simulink model "astrobotics_flowchart"  (R2018a)
settings: Solver=FixedStepDiscrete  StartTime=0.0  StopTime=60  FixedStep=0.1  RelTol=1e-3  EnableMultiTasking=on
settings Model: Creator=alex  LastModifiedBy=alex
settings SolverCC: AutoInsertRateTranBlk=on
settings DataIOCC: LimitDataPoints=on
settings OptimizationCC: LifeSpan=inf
settings DebuggingCC: AllowSymbolicDim=off  SFUnexpectedBacktrackingDiag=warning  SFNoUnconditionalDefaultTransitionDiag=warning  SFExecutionAtInitializationDiag=none
settings CodeAppCC: StateflowObjectComments=on
settings GRTTargetCC: TargetLangStandard=C89/C90 (ANSI)
settings ConfigComp: CovMetricSettings=dw  CovHtmlReporting=on  CovSaveCumulativeToWorkspaceVar=on  CovSaveSingleToWorkspaceVar=on  CovShowResultsExplorer=off  CovExternalEMLEnable=off

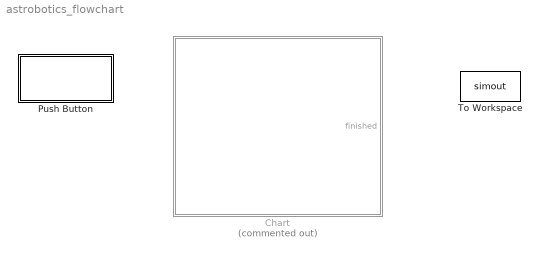
== system astrobotics_flowchart ==
  Chart : Stateflow chart  Commented=on  TreatAsAtomicUnit=on
  Push Button : Subsystem  DialogController=hmiCreateDDGDialog  IsWebBlock=on  mask(MWDashboardBlock){webBlockId=0eb19dcc-6111-4502-8404-cb3df8c1d0d6, webBlockType=pushbutton, ShowInLibBrwoser=on, ShowInitialText=on, HMISrcModelName=astrobotics_flowchart}
      mask prompts: webBlockId "WebBlock Id"; webBlockType "WebBlock Type"; HMISrcModelName "Source Model"
      mask help: SimulinkHMI:dialogs:PushButtonDialogDesc
      mask Help: helpview([docroot '/mapfiles/simulink.map'], 'hmi_push_button')
      mask Display:
      | model = bdroot(gcb);
      | if strcmp(get_param(model,'BlockDiagramType'), 'library')
      |     image([(matlabroot) '/toolbox/simulink/hmi/icons/PushButton.png']);
      | end
  To Workspace : ToWorkspace  VariableName=simout  SaveFormat=Timeseries  SampleTime=-1

== system astrobotics_flowchart/Push Button ==

== stateflow chart astrobotics_flowchart/Chart ==
  state start
    entry: state_select = 0;
    state_select = state_select + 1;
    cycles = 0;
    finished = false;
  state deposit_material
    entry: state_select = 4;
    cycles = cycles + 1;
    state_select = 1;
    if cycles == 5
    state_select = 5;
    end
  state drive_out %State Name
    entry: state_select = 1; % entry action
    state_select = state_select + 1;
    % during:
  state excavate
    entry: state_select = 2;
    state_select = state_select + 1;
  state drive_in
    entry: state_select = 3;
    state_select = state_select + 1;
  state stop
    entry: state_select = 5;
    finished = true;
  (default) -> start : {state_select = 0;}
  start -> drive_out %State Name : [state_select == 1]
  deposit_material -> stop [order 2] : [state_select == 5]
  deposit_material -> drive_out %State Name [order 1] : [state_select == 1]
  drive_out %State Name -> excavate : [state_select == 2]% [transition condition]{action}
  drive_in -> deposit_material : [state_select ==  4]
  excavate -> drive_in : [state_select == 3]
  data: finished output; cycles local; state_select local int32
